simulink model "modelo_deadBeat"  (R2021a)
settings: Solver=VariableStepAuto  StartTime=0.0  StopTime=10.0  RelTol=1e-3
values from neighbouring files (symbols this model uses):
  Cd = minreal(F/(Pd-F*Pd))    [ScriptDeadBeat.m]    (also in scriptPruebaP.m = Cd_p; scriptPruebaPID.m = Cd_pid)
  Crd = Cd    [ScriptDeadBeat.m]    (also in scriptPruebaP.m = Crd_p; scriptPruebaPID.m = Crd_pid)
  P = Km/(Tm*s+1)/(Tf*s+1)    [ScriptDeadBeat.m]    (also in scriptPrueba.m = 0.03/(1+0.07*s)/(1+0.2*s); scriptPruebaP.m = 0.03/(1+0.07*s)/(1+0.2*s); scriptPruebaPID.m = 0.03/(1+0.07*s)/(1+0.2*s))
  ts = Ts    (= 4)    [ScriptDeadBeat.m]    (also in scriptPrueba.m = 0.025; scriptPruebaP.m = 0.025; scriptPruebaPID.m = 0.015)
settings Model: Creator=ferna  LastModifiedBy=quint

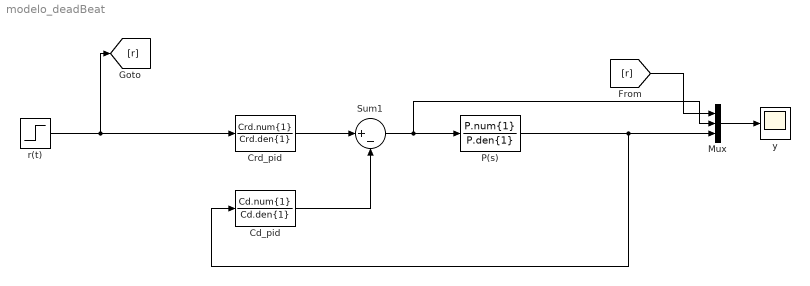
== system modelo_deadBeat ==
  Cd_pid : DiscreteTransferFcn  Numerator=Cd.num{1}  Denominator=Cd.den{1}  SampleTime=ts
  Crd_pid : DiscreteTransferFcn  Numerator=Crd.num{1}  Denominator=Crd.den{1}  SampleTime=ts
  Mux : Mux  Inputs=3
  P(s) : TransferFcn  Numerator=P.num{1}  Denominator=P.den{1}
  Sum1 : Sum  Inputs=|+-
  r(t) : Step  Time=0  SampleTime=0
  y : Scope
  wires:
  [r] -> Mux/1
  Mux/1 -> y/1
  Crd_pid/1 -> Sum1/1
  r(t)/1 -> Crd_pid/1, [r]
  P(s)/1 -> Cd_pid/1, Mux/3
  Sum1/1 -> Mux/2, P(s)/1
  Cd_pid/1 -> Sum1/2
